simulink model "ctrl_HSMBObserver"  (R2015a)
settings: Solver=ode3  StartTime=0.0  StopTime=inf  FixedStep=0.01  RelTol=1e-3
values from neighbouring files (symbols this model uses):
  C = [C1;C2;C3;C4;C5;C6]    [initfile.m]    (also in thrustallocationQuadraticFixed.m)
  D = 3.0/100    (= 0.03)    [initfile.m]    (also in thrustallocationQuadraticFixed.m = 0.0411111111111)
  eps_c = 5    [initfile.m]
  epsilon = 0.5    [initfile.m]    (also in thrustallocationPseudo.m = u(10); thrustallocationQuadraticFixed.m = u(10))
  hd = c2d(H1,0.01,'foh')    [initfile.m]
  hd2 = c2d(H2,0.01,'zoh')    [initfile.m]
  I_s = 25000 /747225    (= 0.0334571246947)    [initfile.m]
  k_cc = 1    [initfile.m]
  K_omega = 0.3    [initfile.m]
  K_q1f = 0.0113    [initfile.m]
  K_q1r = K_q1f    (= 0.0113)    [initfile.m]
  K_q2f = 0.0117    [initfile.m]
  K_q2r = K_q2f    (= 0.0117)    [initfile.m]
  K_q3f = 0.0113    [initfile.m]
  K_q3r = K_q3f    (= 0.0113)    [initfile.m]
  K_q4f = 0.0169    [initfile.m]
  K_q4r = K_q4f    (= 0.0169)    [initfile.m]
  K_q5f = 0.0144    [initfile.m]
  K_q5r = K_q5f    (= 0.0144)    [initfile.m]
  K_q6f = 0.0168    [initfile.m]
  K_q6r = K_q6f    (= 0.0168)    [initfile.m]
  K_T1f = 0.3763    [initfile.m]
  K_T1r = K_T1f    (= 0.3763)    [initfile.m]
  K_T2f = 0.3901    [initfile.m]
  K_T2r = K_T2f    (= 0.3901)    [initfile.m]
  K_T3f = 0.3776    [initfile.m]
  K_T3r = K_T3f    (= 0.3776)    [initfile.m]
  K_T4f = 0.5641    [initfile.m]
  K_T4r = K_T4f    (= 0.5641)    [initfile.m]
  K_T5f = 0.4799    [initfile.m]
  K_T5r = K_T5f    (= 0.4799)    [initfile.m]
  K_T6f = 0.5588    [initfile.m]
  K_T6r = K_T6f    (= 0.5588)    [initfile.m]
  Kp = 3.3    [initfile.m]
  Max_Acceleration = 5    [initfile.m]
  Max_rotation = 12*sqrt(lambda)    [initfile.m]
  Max_thrust = 1.5    [initfile.m]
  Min_thrust = -0.8    [initfile.m]
  n_c = 5    [initfile.m]
  n_max = 152    [initfile.m]
  p_cc = 0.5    [initfile.m]
  pwm_thr1_backward = coeffvalues(ForceToPWM)    [initfile.m]
  pwm_thr1_forward = coeffvalues(ForceToPWM)    [initfile.m]
  pwm_thr2_backward = coeffvalues(ForceToPWM)    [initfile.m]
  pwm_thr2_forward = coeffvalues(ForceToPWM)    [initfile.m]
  pwm_thr3_backward = coeffvalues(ForceToPWM)    [initfile.m]
  pwm_thr3_forward = coeffvalues(ForceToPWM)    [initfile.m]
  pwm_thr4_backward = coeffvalues(ForceToPWM)    [initfile.m]
  pwm_thr4_forward = coeffvalues(ForceToPWM)    [initfile.m]
  pwm_thr5_backward = coeffvalues(ForceToPWM)    [initfile.m]
  pwm_thr5_forward = coeffvalues(ForceToPWM)    [initfile.m]
  pwm_thr6_backward = coeffvalues(ForceToPWM)    [initfile.m]
  pwm_thr6_forward = coeffvalues(ForceToPWM)    [initfile.m]
  Q_f0 = 0.3    [initfile.m]
  r_cc = 4    [initfile.m]
  Rho = Rho_m    (= 1000)    [initfile.m]
  ts = [-1 0]    [thrustallocationPseudo.m]    (also in thrustallocationQuadraticFixed.m)
undefined symbols (not defined in the file or in its folder): AFB, arm, Att, Control, Damping, FaultDet, Glob, Grip, IntActionType, Mass, NPO, Obs, Omg0_min, Q_max, ReferenceMdl, Sensor, Sim, SwLogic, tau, Thruster, Thruster_lock
libraries: dspmtrx3 x14, marine_gnc x11, simulink_extras x9, dspstat3 x9, simulink x9, dsparch4 x6, dspspect3 x6
(part 3 of 7)

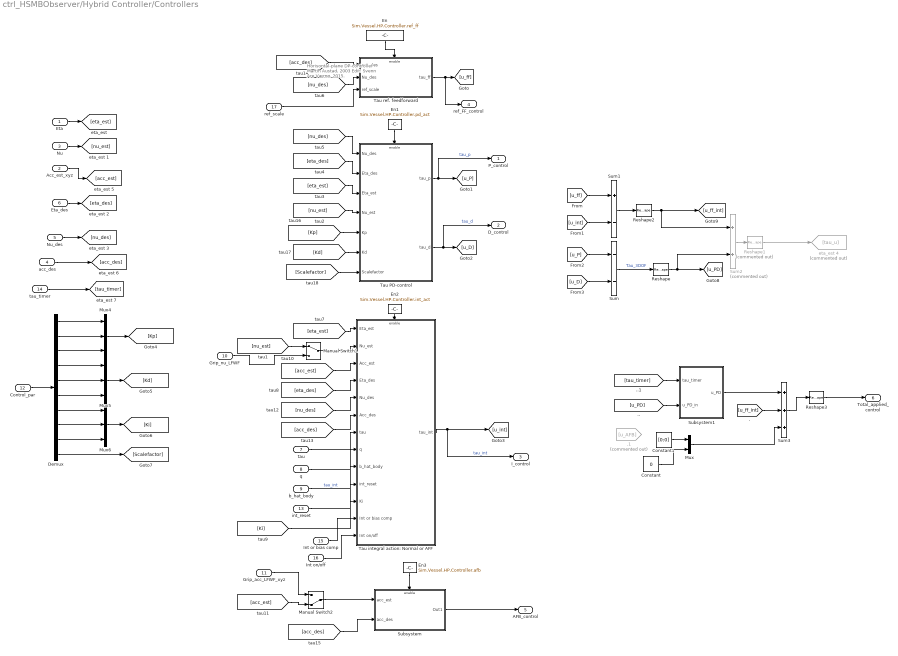
== system ctrl_HSMBObserver/Hybrid Controller/Controllers ==
  note: Horisontal-plane DP-controller
      | Martin Austad, 2003
      |
      | Edit: Svenn Are Værnø, 2015.
  Eta : Inport
  Acc_est_xyz : Inport  Port=2  PortDimensions=3
  Nu : Inport  Port=3
  acc_des : Inport  Port=4
  Nu_des : Inport  Port=5
  Eta_des : Inport  Port=6
  tau : Inport  Port=7
  q : Inport  Port=8
  b_hat_body : Inport  Port=9
  Grip_nu_LFWF : Inport  Port=10
  Grip_acc_LFWF_xyz : Inport  Port=11
  Control_par : Inport  Port=12
  int_reset : Inport  Port=13
  tau_timer : Inport  Port=14
  Int or bias comp : Inport  Port=15
  Int on/off : Inport  Port=16
  ref_scale : Inport  Port=17
  .1 : From  Commented=on  GotoTag=u_AFB
  Constant : Constant  Value=0
  Constant1 : Constant  Value=[0;0]
  Demux : Demux  Outputs=10
  En : Constant  Value=Sim.Vessel.HP.Controller.ref_ff
  En1 : Constant  Value=Sim.Vessel.HP.Controller.pd_act
  En2 : Constant  Value=Sim.Vessel.HP.Controller.int_act
  En3 : Constant  Value=Sim.Vessel.HP.Controller.afb
  Manual Switch1 : ManualSwitch
  Manual Switch2 : ManualSwitch  CurrentSetting=0
  Mux : Mux  Inputs=2
  Mux4 : Mux  Inputs=3
  Mux5 : Mux  Inputs=3
  Mux6 : Mux  Inputs=3
  Reshape : Reshape
  Reshape1 : Reshape  Commented=on
  Reshape2 : Reshape
  Reshape3 : Reshape
  Subsystem : Subsystem
  Subsystem1 : Subsystem
  Sum : Sum  Inputs=--  SaturateOnIntegerOverflow=on
  Sum1 : Sum  Inputs=+-  SaturateOnIntegerOverflow=on
  Sum2 : Sum  Commented=on  SaturateOnIntegerOverflow=on
  Sum3 : Sum  Inputs=+++  SaturateOnIntegerOverflow=on
  Tau PD-control : Subsystem
  Tau integral action: Normal or AFF : Subsystem
  Tau ref. feedforward : Subsystem
  eta_est 4 : Goto  Commented=on  GotoTag=tau_u
  P_control : Outport
  D_control : Outport  Port=2
  I_control : Outport  Port=3
  ref_FF_control : Outport  Port=4
  AFB_control : Outport  Port=5
  Total_applied_control : Outport  Port=6
  wires:
  Tau ref. feedforward/1(tau_ff) -> ref_FF_control/1, [u_ff]
  En/1 -> Tau ref. feedforward/Enable
  En2/1 -> Tau integral action: Normal or AFF/Enable
  En1/1 -> Tau PD-control/Enable
  Reshape/1 -> [u_PD], Sum2/2
  Eta/1 -> [eta_est]
  Nu/1 -> [nu_est]
  [nu_est] -> Tau PD-control/4(Nu_est)
  [eta_est] -> Tau PD-control/3(Eta_est)
  Nu_des/1 -> [nu_des]
  Eta_des/1 -> [eta_des]
  [eta_des] -> Tau PD-control/2(Eta_des)
  [nu_des] -> Tau PD-control/1(Nu_des)
  [nu_des] -> Tau ref. feedforward/2(Nu_des)
  Sum/1 -> Reshape/1  "Tau_3DOF"
  Sum2/1 -> Reshape1/1
  Reshape1/1 -> eta_est 4/1
  Reshape2/1 -> [u_ff_int], Sum2/1
  Sum1/1 -> Reshape2/1
  Tau PD-control/1(tau_p) -> P_control/1, [u_P]  "tau_p"
  Tau PD-control/2(tau_d) -> D_control/1, [u_D]  "tau_d"
  [u_ff] -> Sum1/1
  [u_int] -> Sum1/2
  [u_P] -> Sum/1
  [u_D] -> Sum/2
  Grip_nu_LFWF/1 -> Manual Switch1/2
  [nu_est] -> Manual Switch1/1
  Acc_est_xyz/1 -> [acc_est]
  En3/1 -> Subsystem/Enable
  Subsystem/1(Out1) -> AFB_control/1
  [acc_est] -> Manual Switch2/2
  Grip_acc_LFWF_xyz/1 -> Manual Switch2/1
  Manual Switch2/1 -> Subsystem/1(acc_est)
  [eta_est] -> Tau integral action: Normal or AFF/1(Eta_est)
  Manual Switch1/1 -> Tau integral action: Normal or AFF/2(Nu_est)
  [acc_est] -> Tau integral action: Normal or AFF/3(Acc_est)
  [eta_des] -> Tau integral action: Normal or AFF/4(Eta_des)
  tau/1 -> Tau integral action: Normal or AFF/7(tau)
  acc_des/1 -> [acc_des]
  Tau integral action: Normal or AFF/1(tau_int) -> I_control/1, [u_int]  "tau_int"
  [acc_des] -> Tau ref. feedforward/1(acc_des)
  [nu_des] -> Tau integral action: Normal or AFF/5(Nu_des)
  q/1 -> Tau integral action: Normal or AFF/8(q)
  b_hat_body/1 -> Tau integral action: Normal or AFF/9(b_hat_body)  "tau_int"
  [acc_des] -> Tau integral action: Normal or AFF/6(Acc_des)
  Control_par/1 -> Demux/1
  Demux/1 -> Mux4/1
  Demux/2 -> Mux4/2
  Demux/3 -> Mux4/3
  Demux/4 -> Mux5/1
  Demux/5 -> Mux5/2
  Demux/6 -> Mux5/3
  Demux/7 -> Mux6/1
  Demux/8 -> Mux6/2
  Demux/9 -> Mux6/3
  Mux4/1 -> [Kp]
  Mux5/1 -> [Kd]
  Mux6/1 -> [Ki]
  Demux/10 -> [Scalefactor]
  int_reset/1 -> Tau integral action: Normal or AFF/10(int_reset)
  [Ki] -> Tau integral action: Normal or AFF/11(Ki)
  [acc_des] -> Subsystem/2(acc_des)
  [Scalefactor] -> Tau PD-control/7(Scalefactor)
  [Kd] -> Tau PD-control/6(Kd)
  [Kp] -> Tau PD-control/5("Kp ")
  Sum3/1 -> Reshape3/1
  [u_ff_int] -> Sum3/2
  [u_PD] -> Subsystem1/2(u_PD_in)
  [tau_timer] -> Subsystem1/1(tau_timer)
  Constant/1 -> Mux/2
  Mux/1 -> Sum3/3
  Subsystem1/1(u_PD) -> Sum3/1
  Reshape3/1 -> Total_applied_control/1
  tau_timer/1 -> [tau_timer]
  Constant1/1 -> Mux/1
  Int or bias comp/1 -> Tau integral action: Normal or AFF/12(Int or bias comp)
  Int on/off/1 -> Tau integral action: Normal or AFF/13(Int on/off)
  ref_scale/1 -> Tau ref. feedforward/3(ref_scale)

== system ctrl_HSMBObserver/Hybrid Controller/Fault Detection (freeze) ==
  note: Fault detection
      | Variance testing MarReg compendium p. 153
      | SA Værnø and AH Brodtkorb fall 2015
  Eta_6DOFmeas : Inport
  Buffer : Buffer  N=FaultDet.n  V=FaultDet.ovl  ic=0.5  TreatMby1Signals=One channel
  If : If  NumInputs=2  IfExpression=u1 == u2
  If Action Subsystem : Subsystem  TreatAsAtomicUnit=on
  If Action Subsystem1 : Subsystem  TreatAsAtomicUnit=on
  Mean : dspstat3/Mean  run=off  reset_popup=None  InputProcessing=Columns as channels (frame based)  directionMode=Each column  dimension=1  treatSBRowAsCol=on  roiEnable=off  roiType=Rectangles  roiPortion=Entire ROI  roiOutput=Individual statistics for each ROI  roiFlag=off  outputDataTypeStr=Inherit: Same as accumulator  outputLastDataTypeStr=Inherit: Same as accumulator  outputMin=[]  outputMax=[]  roundingMode=Floor  overflowMode=off
  Merge : Merge
  Merge1 : Merge
  Rate Transition2 : RateTransition  Deterministic=off
  Reshape : Reshape
  Selector : Selector  InputPortWidth=6  Indices=[1]
  Unit Delay : UnitDelay  SampleTime=-1
  Zero-Order Hold3 : ZeroOrderHold  SampleTime=1/FaultDet.Fs
  fault : Outport
  pos_injection : Outport  Port=2
  wires:
  Selector/1 -> Zero-Order Hold3/1
  Eta_6DOFmeas/1 -> Selector/1
  If/1 -> If Action Subsystem/Action
  Unit Delay/1 -> If/1
  If/2 -> If Action Subsystem1/Action
  If Action Subsystem1/1(faultID) -> Merge/2
  Merge/1 -> fault/1
  If Action Subsystem/1(faultID) -> Merge/1
  Merge1/1 -> pos_injection/1
  If Action Subsystem/2(pos_inject) -> Merge1/1
  If Action Subsystem1/2(pos_inject) -> Merge1/2
  Rate Transition2/1 -> If/2, Unit Delay/1
  Buffer/1 -> Reshape/1
  Zero-Order Hold3/1 -> Buffer/1
  Reshape/1 -> Mean/1
  Mean/1 -> Rate Transition2/1

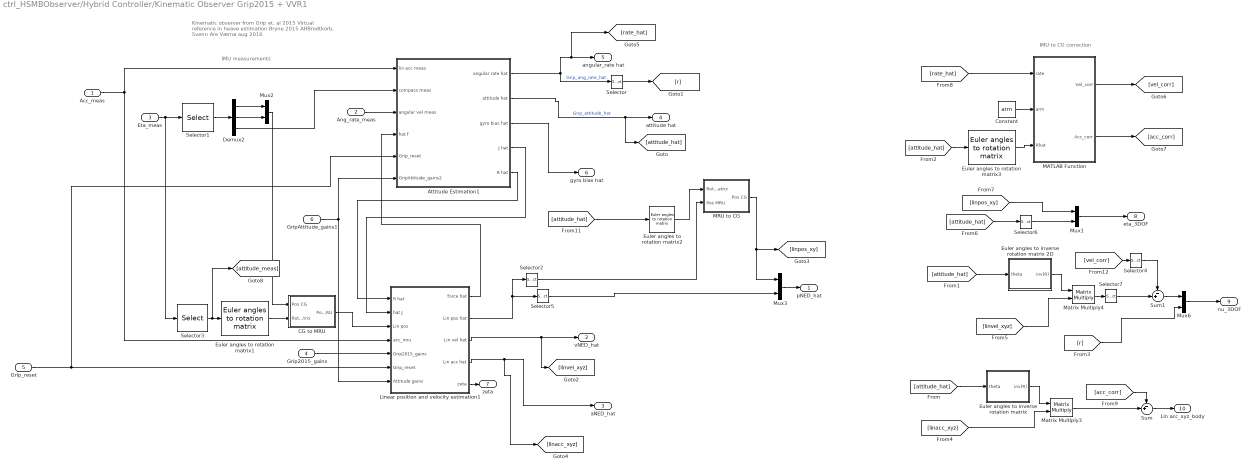
== system ctrl_HSMBObserver/Hybrid Controller/Kinematic Observer Grip2015 + VVR1 ==
  note: IMU to CG correction
  note: Kinematic observer from Grip et. al 2015
      | Virtual reference in heave estimation Bryne 2015
      | AHBrodtkorb, Svenn Are Værnø aug 2016
  note: IMU measurements
  Acc_meas : Inport
  Ang_rate_meas : Inport  Port=2
  Eta_meas : Inport  Port=3
  Grip2015_gains : Inport  Port=4
  Grip_reset : Inport  Port=5
  GripAttitude_gains1 : Inport  Port=6
  Attitude Estimation1 : Subsystem
  CG to MRU : Subsystem
  Constant : Constant  Value=arm
  Demux2 : Demux  Outputs=3
  Euler angles to inverse rotation matrix : Subsystem  AncestorBlock=|  mask(Rbn){}
      | marine_gnc/Models/ Kinematics/Euler angles to
      | inverse rotation
      | matrix
      mask help:
      | Calculate the rotation matrix from NED coordinates to Body coordinates.
      |
      | Input: Theta = [phi, theta, psi]'
      |
      | Output: inv(Rzyx) (3x3)
      mask Help:
      | Calculate the rotation matrix from NED coordinates to Body coordinates.
      | 
      | Input: Theta = [phi, theta, psi]'
      | 
      | Output: inv(Rzyx) (3x3)
  Euler angles to inverse rotation matrix 2D : Subsystem  AncestorBlock=|  mask(Rbn){}
      | marine_gnc/Models/ Kinematics/Euler angles to
      | inverse rotation
      | matrix
      mask help:
      | Calculate the rotation matrix from NED coordinates to Body coordinates.
      |
      | Input: Theta = [phi, theta, psi]'
      |
      | Output: inv(Rzyx) (3x3)
      mask Help:
      | Calculate the rotation matrix from NED coordinates to Body coordinates.
      | 
      | Input: Theta = [phi, theta, psi]'
      | 
      | Output: inv(Rzyx) (3x3)
  Euler angles to rotation matrix1 : marine_gnc/Models/ Kinematics/Euler angles to rotation matrix
  Euler angles to rotation matrix2 : marine_gnc/Models/ Kinematics/Euler angles to rotation matrix
  Euler angles to rotation matrix3 : marine_gnc/Models/ Kinematics/Euler angles to rotation matrix
  Linear position and velocity estimation1 : Subsystem
  MATLAB Function : MATLAB Function  TreatAsAtomicUnit=on
  MRU to CG : Subsystem
  Matrix Multiply3 : Product  Multiplication=Matrix(*)
  Matrix Multiply4 : Product  Multiplication=Matrix(*)
  Mux{1..3,6} (4 alike) : Mux  Inputs=2
  Selector : Selector  InputPortWidth=3  Indices=[3]
  Selector1 : Selector  InputPortWidth=6  Indices=[1 2 6]
  Selector2 : Selector  InputPortWidth=3  Indices=[1 2]
  Selector3 : Selector  InputPortWidth=6  Indices=[4 5 6]
  Selector4 : Selector  InputPortWidth=3  Indices=[1 2]
  Selector5 : Selector  InputPortWidth=3  Indices=[3]
  Selector6 : Selector  InputPortWidth=3  Indices=[3]
  Selector7 : Selector  InputPortWidth=3  Indices=[1 2]
  Sum : Sum  Inputs=-+|
  Sum1 : Sum  Inputs=-+|
  pNED_hat : Outport
  vNED_hat : Outport  Port=2
  aNED_hat : Outport  Port=3
  attitude hat : Outport  Port=4
  angular_rate hat : Outport  Port=5
  gyro bias hat : Outport  Port=6
  zeta : Outport  Port=7
  eta_3DOF : Outport  Port=8
  nu_3DOF : Outport  Port=9
  Lin acc_xyz_body : Outport  Port=10
  wires:
  Selector1/1 -> Demux2/1
  Ang_rate_meas/1 -> Attitude Estimation1/3(angular vel meas)
  Demux2/1 -> Mux2/1
  Demux2/2 -> Mux2/2
  Mux2/1 -> CG to MRU/1(Pos CG)
  Mux3/1 -> pNED_hat/1
  Linear position and velocity estimation1/4(Lin acc hat) -> [linacc_xyz], aNED_hat/1
  Linear position and velocity estimation1/3(Lin vel hat) -> [linvel_xyz], vNED_hat/1
  Linear position and velocity estimation1/2(Lin pos hat) -> Selector5/1, Selector2/1
  Selector/1 -> [r]
  Demux2/3 -> Attitude Estimation1/2(compass meas)
  MRU to CG/1(Pos CG) -> Mux3/1, [linpos_xy]
  Attitude Estimation1/2(attitude hat) -> [attitude_hat], attitude hat/1  "Grip_attitude_hat"
  Attitude Estimation1/1(angular rate hat) -> [rate_hat], angular_rate hat/1, Selector/1  "Grip_ang_rate_hat"
  Attitude Estimation1/3(gyro bias hat) -> gyro bias hat/1
  Linear position and velocity estimation1/5(zeta) -> zeta/1
  Selector5/1 -> Mux3/2
  [linacc_xyz] -> Matrix Multiply3/2
  Euler angles to inverse rotation matrix/1(inv(R)) -> Matrix Multiply3/1
  [attitude_hat] -> Euler angles to inverse rotation matrix/1(theta)
  [linvel_xyz] -> Matrix Multiply4/2
  Euler angles to inverse rotation matrix 2D/1(inv(R)) -> Matrix Multiply4/1
  [r] -> Mux6/2
  [attitude_hat] -> Euler angles to inverse rotation matrix 2D/1(theta)
  [attitude_hat] -> Selector6/1
  Selector6/1 -> Mux1/2
  [linpos_xy] -> Mux1/1
  Matrix Multiply4/1 -> Selector7/1
  Selector7/1 -> Sum1/2
  Mux6/1 -> nu_3DOF/1
  Mux1/1 -> eta_3DOF/1
  Attitude Estimation1/4(J hat) -> Linear position and velocity estimation1/2(hat J)
  Acc_meas/1 -> Attitude Estimation1/1(lin acc meas), Linear position and velocity estimation1/4(acc_imu)
  Linear position and velocity estimation1/1(force hat) -> Attitude Estimation1/4(hat f)
  Attitude Estimation1/5(R hat) -> Linear position and velocity estimation1/1(R hat)
  Grip2015_gains/1 -> Linear position and velocity estimation1/5(Grip2015_gains)
  Grip_reset/1 -> Linear position and velocity estimation1/6(Grip_reset), Attitude Estimation1/5(Grip_reset)
  Matrix Multiply3/1 -> Sum/2
  GripAttitude_gains1/1 -> Linear position and velocity estimation1/7(Attitude gains), Attitude Estimation1/6(GripAttitude_gains2)
  [attitude_hat] -> Euler angles to rotation matrix2/1
  Euler angles to rotation matrix2/1 -> MRU to CG/1(Rotation matrix)
  Selector2/1 -> MRU to CG/2(Pos MRU)
  Eta_meas/1 -> Selector3/1, Selector1/1
  Euler angles to rotation matrix1/1 -> CG to MRU/2(Rotation matrix)
  CG to MRU/1(Pos MRU) -> Linear position and velocity estimation1/3(Lin pos)
  [attitude_hat] -> Euler angles to rotation matrix3/1
  Euler angles to rotation matrix3/1 -> MATLAB Function/3(Rhat)
  Constant/1 -> MATLAB Function/2(arm)
  [rate_hat] -> MATLAB Function/1(rate)
  MATLAB Function/2(Acc_corr) -> [acc_corr]
  MATLAB Function/1(Vel_corr) -> [vel_corr]
  Sum/1 -> Lin acc_xyz_body/1
  [acc_corr] -> Sum/1
  Sum1/1 -> Mux6/1
  [vel_corr] -> Selector4/1
  Selector4/1 -> Sum1/1
  Selector3/1 -> [attitude_meas], Euler angles to rotation matrix1/1

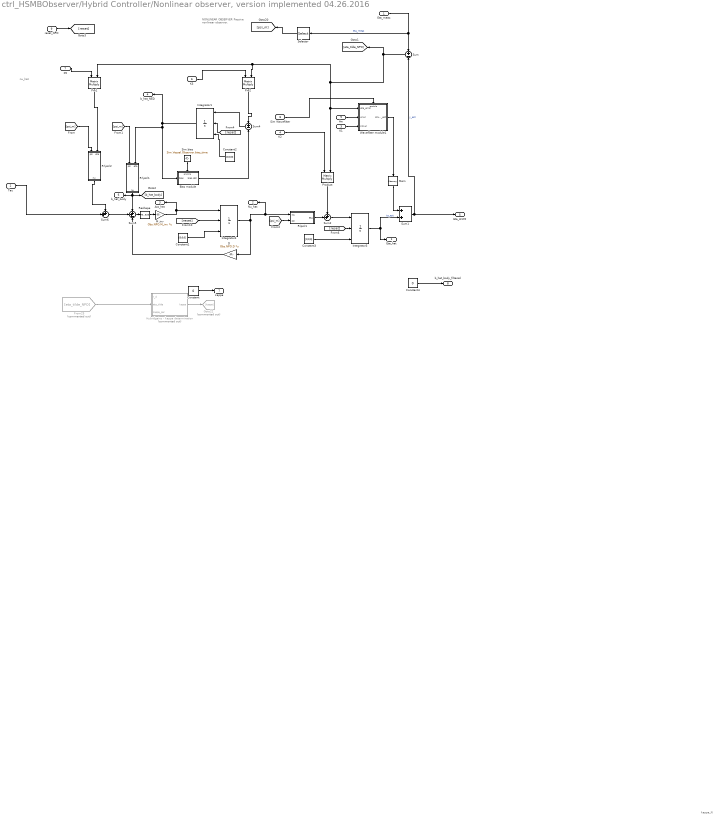
== system ctrl_HSMBObserver/Hybrid Controller/Nonlinear observer, version implemented 04.26.2016 ==
  note: NONLINEAR OBSERVER
      | Passive nonlinear observer.
  note: kappa_N
  note: nu_hat
  Eta_meas : Inport
  Tau : Inport  Port=2
  K1 : Inport  Port=3
  K2 : Inport  Port=4
  Aw : Inport  Port=5
  K3 : Inport  Port=6
  K5 : Inport  Port=7
  Sim Wavefilter : Inport  Port=8
  reset_NPO : Inport  Port=9
  Bias module : Subsystem
  Constant : Constant  Value=0
  Constant1 : Constant  Value=[0;0;0]
  Constant2 : Constant  Value=[0;0;0]
  Constant3 : Constant  Value=[0;0;0]
  Constant4 : Constant  Value=0
  D : Gain  Gain=Obs.NPO.D  Multiplication=Matrix(K*u)  SaturateOnIntegerOverflow=on  OutDataTypeStr=Inherit: Same as input  ParamDataTypeStr=Inherit: Same as input
  From25 : From  Commented=on  GotoTag=eta_tilde_NPO
  Goto22 : Goto  Commented=on  GotoTag=kappa
  Hybridgains - kappa determination : Subsystem  Commented=on
  Integrator1 : Integrator  ExternalReset=either  InitialConditionSource=external
  Integrator3 : Integrator  ExternalReset=either  InitialConditionSource=external
  Integrator4 : Integrator  ExternalReset=either  InitialConditionSource=external
  M_inv : Gain  Gain=Obs.NPO.M_inv  Multiplication=Matrix(K*u)  SaturateOnIntegerOverflow=on  OutDataTypeStr=Inherit: Same as input  ParamDataTypeStr=Inherit: Same as input
  Mem : Memory
  Pro1 : Product  Multiplication=Matrix(*)  SaturateOnIntegerOverflow=on  OutDataTypeStr=Inherit: Same as first input
  Pro2 : Product  Multiplication=Matrix(*)  SaturateOnIntegerOverflow=on  OutDataTypeStr=Inherit: Same as first input
  Product : Product  Multiplication=Matrix(*)  SaturateOnIntegerOverflow=on  OutDataTypeStr=Inherit: Same as first input
  R'(psi)1 : Subsystem
  R'(psi)2 : Subsystem
  R(psi)1 : Subsystem
  Reshape : Reshape
  Selector : Selector  InputPortWidth=3  Indices=3
  Sim.bias : Constant  Value=Sim.Vessel.Observer.bias_time
  Sum : Sum  Inputs=+-  SaturateOnIntegerOverflow=on
  Sum1 : Sum  SaturateOnIntegerOverflow=on
  Sum2 : Sum  Inputs=++|  SaturateOnIntegerOverflow=on
  Sum4 : Sum  Inputs=+-  SaturateOnIntegerOverflow=on
  Sum5 : Sum  Inputs=++-  SaturateOnIntegerOverflow=on
  Sum6 : Sum  Inputs=++|  SaturateOnIntegerOverflow=on
  Wavefilter module1 : Subsystem
  Eta_hat : Outport  InitialOutput=0
  Nu_hat : Outport  Port=2  InitialOutput=0
  Acc_hat : Outport  Port=3  InitialOutput=0
  b_hat_NED : Outport  Port=4  InitialOutput=0
  Eta_LFWF : Outport  Port=5  InitialOutput=0
  b_hat_body : Outport  Port=6  PortDimensions=3  InitialOutput=0
  kappa : Outport  Port=7  InitialOutput=0
  b_hat_body_filtered : Outport  Port=8  InitialOutput=0
  wires:
  Sim.bias/1 -> Bias module/Enable
  Bias module/1(bias.dot) -> Sum4/2
  Sim Wavefilter/1 -> Wavefilter module1/Enable
  Sum1/1 -> Sum/2, Eta_LFWF/1  "y_est"
  Mem/1 -> Sum1/1
  Selector/1 -> [psi_m]
  K1/1 -> Wavefilter module1/3(K1(w))
  Eta_meas/1 -> Selector/1, Sum/1  "eta_meas"
  M_inv/1 -> Integrator4/1, Acc_hat/1
  R'(psi)2/1(nu) -> Sum6/1
  Wavefilter module1/1(Wave_est) -> Mem/1
  Sum6/1 -> Sum5/2
  D/1 -> Sum5/3
  Integrator3/1 -> Sum1/2, Eta_hat/1  "ta_est"
  Aw/1 -> Wavefilter module1/2(A(w))
  Sum/1 -> [eta_tilde_NPO], Pro1/2, Pro2/2, Product/2, Wavefilter module1/1(eta_error)
  R'(psi)1/1(nu) -> [b_hat_body], Sum5/1, b_hat_body/1
  R(psi)1/1(Eta) -> Sum2/2
  K2/1 -> Product/1
  Tau/1 -> Sum6/2
  Pro1/1 -> R'(psi)2/2(eta)
  Pro2/1 -> Sum4/1
  Product/1 -> Sum2/1
  K5/1 -> Pro1/1
  [psi_m] -> R'(psi)2/1(psi)
  [psi_m] -> R'(psi)1/1(psi)
  [psi_m] -> R(psi)1/2(psi)
  Reshape/1 -> M_inv/1
  Sum5/1 -> Reshape/1
  From25/1 -> Hybridgains - kappa determination/2(eta_tilde)
  Hybridgains - kappa determination/1(kappa) -> Goto22/1
  reset_NPO/1 -> [reset]
  [reset] -> Integrator4/2
  Constant1/1 -> Integrator4/3
  Integrator4/1 -> Nu_hat/1, R(psi)1/1(Nu), D/1
  Sum2/1 -> Integrator3/1
  [reset] -> Integrator1/2
  Constant2/1 -> Integrator1/3
  Sum4/1 -> Integrator1/1
  Integrator1/1 -> Bias module/1(bias), R'(psi)1/2(eta), b_hat_NED/1
  [reset] -> Integrator3/2
  Constant3/1 -> Integrator3/3
  K3/1 -> Pro2/1
  Constant/1 -> kappa/1
  Constant4/1 -> b_hat_body_filtered/1

== system ctrl_HSMBObserver/Hybrid Controller/Peak Frequency FFT ==
  Eta_6DOF : Inport
  CalmWater choose PID1 : Subsystem
  Memory : Memory  X0=Control.SA.init_wp  InheritSampleTime=on
  estimate w_p : Subsystem
  hat_wp : Outport
  wires:
  Eta_6DOF/1 -> estimate w_p/1(eta_6DOF)
  Memory/1 -> hat_wp/1
  estimate w_p/1(w_p) -> CalmWater choose PID1/1(wp)
  CalmWater choose PID1/1(wp_out) -> Memory/1

== system ctrl_HSMBObserver/Hybrid Controller/Reference filter ==
  eta_d : Inport
  eta : Inport  Port=2
  PDF filter gains : Inport  Port=3
  Constant{,1..3} (4 alike) : Constant  Value=[0,0,0]
  Demux3 : Demux  Outputs=5
  Mux : Mux  Inputs=2
  Mux1 : Mux
  Scope : Scope
  Scope1 : Scope
  Subsystem : Subsystem
  Switch : Switch  Criteria=u2 > Threshold
  Switch1 : Switch  Criteria=u2 > Threshold
  Switch2 : Switch  Criteria=u2 > Threshold
  eta_c_scope1 : Scope
  eta_d1 : InportShadow
  eta_d_scpoe : Scope
  eta_f_scope : Scope
  eta_scope : Scope
  eta_tot_scop : Scope
  eta_d_f : Outport
  v_d_f : Outport  Port=2
  v_dd_f : Outport  Port=3
  wires:
  Switch/1 -> eta_tot_scop/1, eta_d_f/1
  Switch1/1 -> v_d_f/1
  Switch2/1 -> v_dd_f/1
  [enable] -> Switch/2
  [enable] -> Switch1/2
  [enable] -> Switch2/2
  eta_d/1 -> eta_d_scpoe/1, Mux/2, Switch/3
  Constant2/1 -> Switch1/3
  Constant3/1 -> Switch2/3
  eta_d1/1 -> Subsystem/1(eta_d)
  Subsystem/2(v_d_f) -> Switch1/1, Scope/1
  Subsystem/3(v_dd_f) -> Switch2/1, Scope1/1
  eta/1 -> eta_scope/1, Subsystem/2(eta1)
  Constant1/1 -> Subsystem/4(v_d)
  Constant/1 -> Subsystem/3(v_d_d)
  Mux/1 -> eta_c_scope1/1
  Subsystem/1(eta_d_f) -> Mux/1, Switch/1, eta_f_scope/1
  PDF filter gains/1 -> Demux3/1
  Demux3/1 -> Mux1/1
  Demux3/2 -> Mux1/2
  Demux3/3 -> Mux1/3
  Demux3/4 -> Mux1/4
  Mux1/1 -> [filter_gains]
  Demux3/5 -> [enable]
  [filter_gains] -> Subsystem/5(filter_gains)

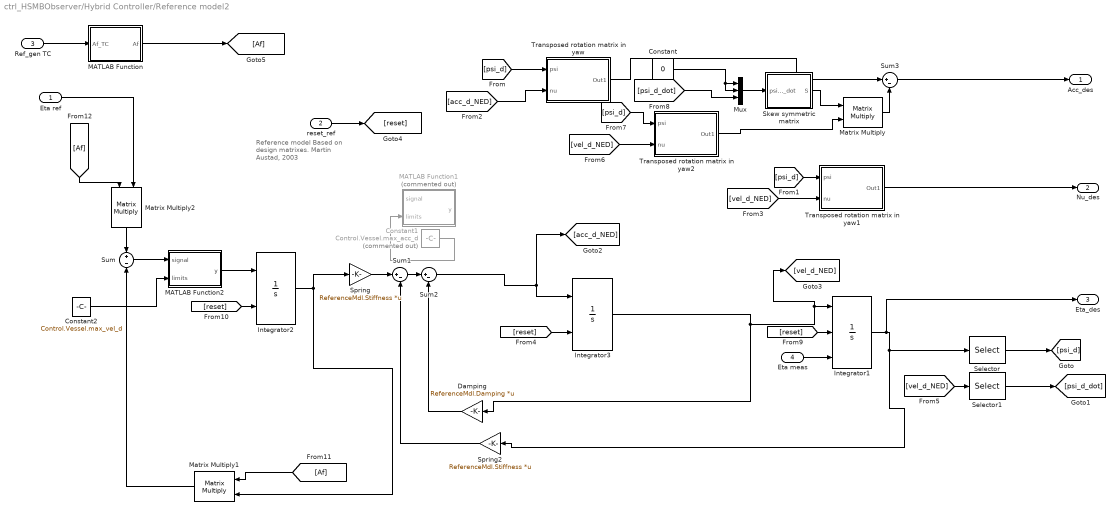
== system ctrl_HSMBObserver/Hybrid Controller/Reference model2 ==
  note: Reference model
      | Based on design matrixes.
      | Martin Austad, 2003
  Eta ref : Inport
  reset_ref : Inport  Port=2
  Ref_gen TC : Inport  Port=3
  Eta meas : Inport  Port=4
  Constant : Constant  Value=0
  Constant1 : Constant  Commented=on  Value=Control.Vessel.max_acc_d
  Constant2 : Constant  Value=Control.Vessel.max_vel_d
  Damping : Gain  Gain=ReferenceMdl.Damping  Multiplication=Matrix(K*u)  SaturateOnIntegerOverflow=on  OutDataTypeStr=Inherit: Same as input  ParamDataTypeStr=Inherit: Same as input
  Integrator1 : Integrator  ExternalReset=either  InitialConditionSource=external
  Integrator2 : Integrator  ExternalReset=either  InitialCondition=[0 0 0]
  Integrator3 : Integrator  ExternalReset=either  InitialCondition=[0 0 0]
  MATLAB Function : MATLAB Function  TreatAsAtomicUnit=on
  MATLAB Function1 : MATLAB Function  Commented=on  TreatAsAtomicUnit=on
  MATLAB Function2 : MATLAB Function  TreatAsAtomicUnit=on
  Matrix Multiply : Product  Multiplication=Matrix(*)
  Matrix Multiply1 : Product  Multiplication=Matrix(*)
  Matrix Multiply2 : Product  Multiplication=Matrix(*)
  Mux : Mux  Inputs=3
  Selector : Selector  InputPortWidth=3  Indices=[3]
  Selector1 : Selector  InputPortWidth=3  Indices=[3]
  Skew symmetric matrix : Subsystem
  Spring : Gain  Gain=ReferenceMdl.Stiffness  Multiplication=Matrix(K*u)  SaturateOnIntegerOverflow=on  OutDataTypeStr=Inherit: Same as input  ParamDataTypeStr=Inherit: Same as input
  Spring2 : Gain  Gain=ReferenceMdl.Stiffness  Multiplication=Matrix(K*u)  SaturateOnIntegerOverflow=on  OutDataTypeStr=Inherit: Same as input  ParamDataTypeStr=Inherit: Same as input
  Sum : Sum  Inputs=+|-  SaturateOnIntegerOverflow=on
  Sum1 : Sum  Inputs=|+-  SaturateOnIntegerOverflow=on
  Sum2 : Sum  Inputs=|+-  SaturateOnIntegerOverflow=on
  Sum3 : Sum  Inputs=|+-
  Transposed rotation matrix in yaw : Subsystem  AncestorBlock="marine_gnc/Models/ Kinematics/Transposed rotation  matrix in yaw"
      mask help:
      | b = R'(psi)* a
      |
      | where
      |
      | input 1:    psi
      | input 2:    a - vector dim 3
      | output 1:  b - vector dim 3
      mask Display:
      | port_label('output', 1, 'R''(psi)*v')
      | port_label('input', 1, 'psi')
      | port_label('input', 2, 'v')
  Transposed rotation matrix in yaw1 : Subsystem  AncestorBlock="marine_gnc/Models/ Kinematics/Transposed rotation  matrix in yaw"
      mask help:
      | b = R'(psi)* a
      |
      | where
      |
      | input 1:    psi
      | input 2:    a - vector dim 3
      | output 1:  b - vector dim 3
      mask Display:
      | port_label('output', 1, 'R''(psi)*v')
      | port_label('input', 1, 'psi')
      | port_label('input', 2, 'v')
  Transposed rotation matrix in yaw2 : Subsystem  AncestorBlock="marine_gnc/Models/ Kinematics/Transposed rotation  matrix in yaw"
      mask help:
      | b = R'(psi)* a
      |
      | where
      |
      | input 1:    psi
      | input 2:    a - vector dim 3
      | output 1:  b - vector dim 3
      mask Display:
      | port_label('output', 1, 'R''(psi)*v')
      | port_label('input', 1, 'psi')
      | port_label('input', 2, 'v')
  Acc_des : Outport
  Nu_des : Outport  Port=2
  Eta_des : Outport  Port=3
  wires:
  Matrix Multiply2/1 -> Sum/1
  Sum/1 -> MATLAB Function2/1(signal)
  Integrator2/1 -> Matrix Multiply1/2, Spring/1
  Matrix Multiply1/1 -> Sum/2
  Spring/1 -> Sum1/1
  Sum1/1 -> Sum2/1
  Integrator1/1 -> Spring2/1, Selector/1, Eta_des/1
  Spring2/1 -> Sum1/2
  Damping/1 -> Sum2/2
  Selector/1 -> [psi_d]
  Transposed rotation matrix in yaw/1(Out1) -> Sum3/1
  [psi_d] -> Transposed rotation matrix in yaw1/1(psi)
  [psi_d] -> Transposed rotation matrix in yaw/1(psi)
  Selector1/1 -> [psi_d_dot]
  [acc_d_NED] -> Transposed rotation matrix in yaw/2(nu)
  [vel_d_NED] -> Transposed rotation matrix in yaw1/2(nu)
  [vel_d_NED] -> Selector1/1
  [psi_d] -> Transposed rotation matrix in yaw2/1(psi)
  [vel_d_NED] -> Transposed rotation matrix in yaw2/2(nu)
  Transposed rotation matrix in yaw2/1(Out1) -> Matrix Multiply/2
  Skew symmetric matrix/1(S) -> Matrix Multiply/1
  Matrix Multiply/1 -> Sum3/2
  [psi_d_dot] -> Mux/3
  Mux/1 -> Skew symmetric matrix/1(psi_d_dot)
  Constant/1 -> Mux/1, Mux/2
  Eta ref/1 -> Matrix Multiply2/2
  reset_ref/1 -> [reset]
  [reset] -> Integrator3/2
  [reset] -> Integrator1/2
  [reset] -> Integrator2/2
  [Af] -> Matrix Multiply1/1
  Ref_gen TC/1 -> MATLAB Function/1(Af_TC)
  MATLAB Function/1(Af) -> [Af]
  Eta meas/1 -> Integrator1/3
  [Af] -> Matrix Multiply2/1
  Transposed rotation matrix in yaw1/1(Out1) -> Nu_des/1
  Sum3/1 -> Acc_des/1
  Constant1/1 -> MATLAB Function1/2(limits)
  Sum2/1 -> Integrator3/1, [acc_d_NED]
  Integrator3/1 -> [vel_d_NED], Integrator1/1, Damping/1
  Constant2/1 -> MATLAB Function2/2(limits)
  MATLAB Function2/1(y) -> Integrator2/1

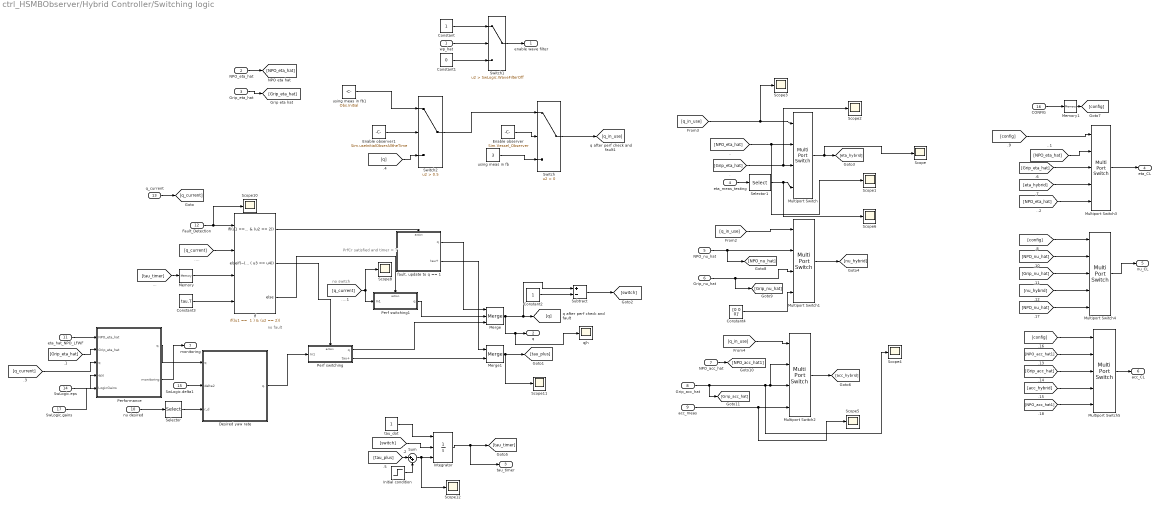
== system ctrl_HSMBObserver/Hybrid Controller/Switching logic ==
  note: PrfCr satisfied and timer = T
  note: no switch
  note: no fault
  wp_hat : Inport
  NPO_eta_hat : Inport  Port=2
  Grip_eta_hat : Inport  Port=3
  eta_meas_testing : Inport  Port=4
  NPO_nu_hat : Inport  Port=5
  Grip_nu_hat : Inport  Port=6
  NPO_acc_hat : Inport  Port=7
  Grip_acc_hat : Inport  Port=8
  acc_meas : Inport  Port=9
  nu desired : Inport  Port=10
  eta_hat_NPO_LFWF : Inport  Port=11
  Fault_Detection : Inport  Port=12
  q_current : Inport  Port=13
  SwLogic.eps : Inport  Port=14
  SwLogic.delta1 : Inport  Port=15
  CONFIG : Inport  Port=16
  SwLogic.gains : Inport  Port=17
  Constant : Constant
  Constant1 : Constant  Value=0
  Constant2 : Constant
  Constant3 : Constant  Value=tau.T
  Constant4 : Constant  Value=[0 0 0]'
  Desired yaw rate : Subsystem
  Enable observer : Constant  Value=Sim.Vessel_Observer
  Enable observer1 : Constant  Value=Sim.useInitialObserAlltheTime
  If : If  NumInputs=4  IfExpression="(u1 ==  1 ) & (u2 == 2)"  ElseIfExpressions="~(u1 ==  1) & ( u3 == u4)"
  Initial condition : Step  Before=tau.T  After=0  SampleTime=0
  Integrator : Integrator  ExternalReset=either  InitialConditionSource=external  LimitOutput=on  UpperSaturationLimit=tau.T  LowerSaturationLimit=0
  Memory : Memory
  Memory1 : Memory  X0=1
  Merge : Merge  Inputs=3
  Merge1 : Merge
  Multiport Switch : MultiPortSwitch
  Multiport Switch1 : MultiPortSwitch
  Multiport Switch2 : MultiPortSwitch
  Multiport Switch3 : MultiPortSwitch  DataPortForDefault=Additional data port  DiagnosticForDefault=None
  Multiport Switch4 : MultiPortSwitch  DataPortForDefault=Additional data port  DiagnosticForDefault=None
  Multiport Switch5 : MultiPortSwitch  DataPortForDefault=Additional data port  DiagnosticForDefault=None
  Perf switching : Subsystem  TreatAsAtomicUnit=on
  Perf switching1 : Subsystem  TreatAsAtomicUnit=on
  Performance : Subsystem
  Scope{,1..6,8,10..12} (11 alike) : Scope
      Scope settings: SaveName=ScopeData50
      Scope1 settings: SaveName=ScopeData51
      Scope10 settings: TimeRange=200  YMin=-1  YMax=1  SaveName=ScopeData153
      Scope11 settings: YMin=0  YMax=3.25e-21  SaveName=ScopeData154
      Scope12 settings: YMin=0  YMax=3.25e-21  SaveName=ScopeData163
      Scope2 settings: YMin=-0.8  YMax=0.4  SaveName=ScopeData52
      Scope3 settings: TimeRange=200  YMin=1  YMax=1  SaveName=ScopeData53
      Scope4 settings: TimeRange=1000  YMin=-0.0006  YMax=0  SaveName=ScopeData101
      Scope5 settings: YMin=-0.008  YMax=0.003  SaveName=ScopeData102
      Scope6 settings: YMin=-0.2  YMax=0  SaveName=ScopeData96
      Scope8 settings: YMin=19  YMax=21  SaveName=ScopeData151
  Selector : Selector  InputPortWidth=3  Indices=[3]
  Selector1 : Selector  InputPortWidth=6  Indices=[1 2 6]
  Subtract : Sum  Inputs=+-
  Sum : Sum  Inputs=|++
  Switch : Switch  Criteria=u2 > Threshold
  Switch1 : Switch  Criteria=u2 > Threshold  Threshold=SwLogic.WaveFilterOff  SaturateOnIntegerOverflow=on
  Switch2 : Switch  Criteria=u2 > Threshold  Threshold=0.5
  "fault, update to q == 1" : Subsystem  TreatAsAtomicUnit=on
  qjh : Scope
      settings: YMin=19  YMax=21  SaveName=ScopeData81
  tau_dot : Constant
  using meas in fb : Constant  Value=3
  using meas in fb1 : Constant  Value=Obs.Initial
  enable wave filter : Outport
  q : Outport  Port=2
  tau_timer : Outport  Port=3
  eta_CL : Outport  Port=4
  nu_CL : Outport  Port=5
  acc_CL : Outport  Port=6
  monitoring : Outport  Port=7
  wires:
  wp_hat/1 -> Switch1/2
  Constant/1 -> Switch1/1
  Constant1/1 -> Switch1/3
  Switch1/1 -> enable wave filter/1
  [NPO_eta_hat] -> Scope1/1, Multiport Switch/2
  [Grip_eta_hat] -> Scope2/1, Multiport Switch/3
  eta_meas_testing/1 -> Selector1/1
  Multiport Switch/1 -> [eta_hybrid], Scope/1
  [q_in_use] -> Multiport Switch1/1
  Multiport Switch1/1 -> [nu_hybrid]
  NPO_nu_hat/1 -> [NPO_nu_hat], Multiport Switch1/2
  Grip_nu_hat/1 -> [Grip_nu_hat], Multiport Switch1/3
  [q_in_use] -> Multiport Switch2/1
  Multiport Switch2/1 -> [acc_hybrid]
  Grip_acc_hat/1 -> [Grip_acc_hat], Scope4/1, Multiport Switch2/2, Multiport Switch2/3
  acc_meas/1 -> Multiport Switch2/4, Scope5/1
  NPO_eta_hat/1 -> [NPO_eta_hat]
  Grip_eta_hat/1 -> [Grip_eta_hat]
  eta_hat_NPO_LFWF/1 -> Performance/1(NPO_eta_hat)
  [Grip_eta_hat] -> Performance/2(Grip_eta_hat)
  Fault_Detection/1 -> Scope10/1, If/1
  If/3 -> Perf switching1/Action
  If/1 -> "fault, update to q == 1"/Action
  If/2 -> Perf switching/Action
  Enable observer/1 -> Switch/2
  using meas in fb/1 -> Switch/3
  q_current/1 -> [q_current]
  [q_current] -> If/2
  Integrator/1 -> tau_timer/1, [tau_timer]
  "fault, update to q == 1"/1(q) -> Merge/1
  Perf switching/1(q) -> Merge/3
  "fault, update to q == 1"/2(tau+) -> Merge1/1
  [tau_timer] -> Memory/1
  Constant3/1 -> If/4
  Desired yaw rate/1(q.) -> Perf switching/1(In1)
  [q_current] -> Perf switching1/1(In1), Scope8/1
  Perf switching1/1(q) -> Merge/2
  Perf switching/2(tau+) -> Merge1/2
  Merge/1 -> qjh/1, q/1, Subtract/1, [q]
  Merge1/1 -> Scope11/1, [tau_plus]
  Memory/1 -> If/3
  tau_dot/1 -> Integrator/1
  Constant2/1 -> Subtract/2
  Subtract/1 -> [switch]
  [switch] -> Integrator/2
  [tau_plus] -> Sum/1
  Initial condition/1 -> Sum/2
  Sum/1 -> Scope12/1, Integrator/3
  [q_in_use] -> Scope3/1, Multiport Switch/1
  Switch/1 -> [q_in_use]
  using meas in fb1/1 -> Switch2/1
  Enable observer1/1 -> Switch2/2
  Switch2/1 -> Switch/1
  [q] -> Switch2/3
  SwLogic.eps/1 -> Performance/4(eps)
  nu desired/1 -> Selector/1
  SwLogic.delta1/1 -> Desired yaw rate/2(delta2)
  [q_current] -> Performance/3(q)
  Performance/1(q.) -> Desired yaw rate/1(q)
  Multiport Switch3/1 -> eta_CL/1
  [NPO_eta_hat] -> Multiport Switch3/2
  [Grip_eta_hat] -> Multiport Switch3/3
  [eta_hybrid] -> Multiport Switch3/4
  Multiport Switch4/1 -> nu_CL/1
  [Grip_nu_hat] -> Multiport Switch4/3
  [NPO_nu_hat] -> Multiport Switch4/2
  [nu_hybrid] -> Multiport Switch4/4
  NPO_acc_hat/1 -> [NPO_acc_hat1]
  [Grip_acc_hat] -> Multiport Switch5/3
  [NPO_acc_hat1] -> Multiport Switch5/2
  [acc_hybrid] -> Multiport Switch5/4
  Multiport Switch5/1 -> acc_CL/1
  Selector/1 -> Desired yaw rate/3(r_d)
  [config] -> Multiport Switch3/1
  [config] -> Multiport Switch4/1
  [config] -> Multiport Switch5/1
  Memory1/1 -> [config]
  CONFIG/1 -> Memory1/1
  [NPO_eta_hat] -> Multiport Switch3/5
  [NPO_nu_hat] -> Multiport Switch4/5
  [NPO_acc_hat1] -> Multiport Switch5/5
  Constant4/1 -> Multiport Switch1/4
  Selector1/1 -> Multiport Switch/4, Scope6/1
  SwLogic.gains/1 -> Performance/5(LogicGains)
  Performance/2(monitoring) -> monitoring/1

== system ctrl_HSMBObserver/Hybrid Controller/[-inf inf] to [-pi pi] ==
  note: x
  note: r
  x [-inf inf] : Inport
  Constant : Constant  Value=2*pi
  Gain : Gain  Gain=pi  SaturateOnIntegerOverflow=on  OutDataTypeStr=Inherit: Same as input  ParamDataTypeStr=Inherit: Same as input
  Math Function : Math  Operator=rem  SaturateOnIntegerOverflow=on
  Saturation : Saturate  UpperLimit=1e10  LowerLimit=-1e10
  Sign : Signum
  Sum : Sum  Inputs=|+-  SaturateOnIntegerOverflow=on
  Sum1 : Sum  Inputs=|++  SaturateOnIntegerOverflow=on
  y [-pi pi] : Outport
  wires:
  x [-inf inf]/1 -> Saturation/1
  Sign/1 -> Gain/1
  Gain/1 -> Sum/2, Sum1/2
  Sum1/1 -> Math Function/1
  Constant/1 -> Math Function/2
  Math Function/1 -> Sum/1
  Sum/1 -> y [-pi pi]/1
  Saturation/1 -> Sum1/1, Sign/1

== system ctrl_HSMBObserver/Hybrid Controller/[-inf inf] to [-pi pi]1 ==
  note: x
  note: r
  x [-inf inf] : Inport
  Constant : Constant  Value=2*pi
  Gain : Gain  Gain=pi  SaturateOnIntegerOverflow=on  OutDataTypeStr=Inherit: Same as input  ParamDataTypeStr=Inherit: Same as input
  Math Function : Math  Operator=rem  SaturateOnIntegerOverflow=on
  Saturation : Saturate  UpperLimit=1e10  LowerLimit=-1e10
  Sign : Signum
  Sum : Sum  Inputs=|+-  SaturateOnIntegerOverflow=on
  Sum1 : Sum  Inputs=|++  SaturateOnIntegerOverflow=on
  y [-pi pi] : Outport
  wires:
  x [-inf inf]/1 -> Saturation/1
  Sign/1 -> Gain/1
  Gain/1 -> Sum/2, Sum1/2
  Sum1/1 -> Math Function/1
  Constant/1 -> Math Function/2
  Math Function/1 -> Sum/1
  Sum/1 -> y [-pi pi]/1
  Saturation/1 -> Sum1/1, Sign/1

== system ctrl_HSMBObserver/Hybrid Controller/[-inf inf] to [-pi pi]2 ==
  note: x
  note: r
  x [-inf inf] : Inport
  Constant : Constant  Value=2*pi
  Gain : Gain  Gain=pi  SaturateOnIntegerOverflow=on  OutDataTypeStr=Inherit: Same as input  ParamDataTypeStr=Inherit: Same as input
  Math Function : Math  Operator=rem  SaturateOnIntegerOverflow=on
  Saturation : Saturate  UpperLimit=1e10  LowerLimit=-1e10
  Sign : Signum
  Sum : Sum  Inputs=|+-  SaturateOnIntegerOverflow=on
  Sum1 : Sum  Inputs=|++  SaturateOnIntegerOverflow=on
  y [-pi pi] : Outport
  wires:
  x [-inf inf]/1 -> Saturation/1
  Sign/1 -> Gain/1
  Gain/1 -> Sum/2, Sum1/2
  Sum1/1 -> Math Function/1
  Constant/1 -> Math Function/2
  Math Function/1 -> Sum/1
  Sum/1 -> y [-pi pi]/1
  Saturation/1 -> Sum1/1, Sign/1

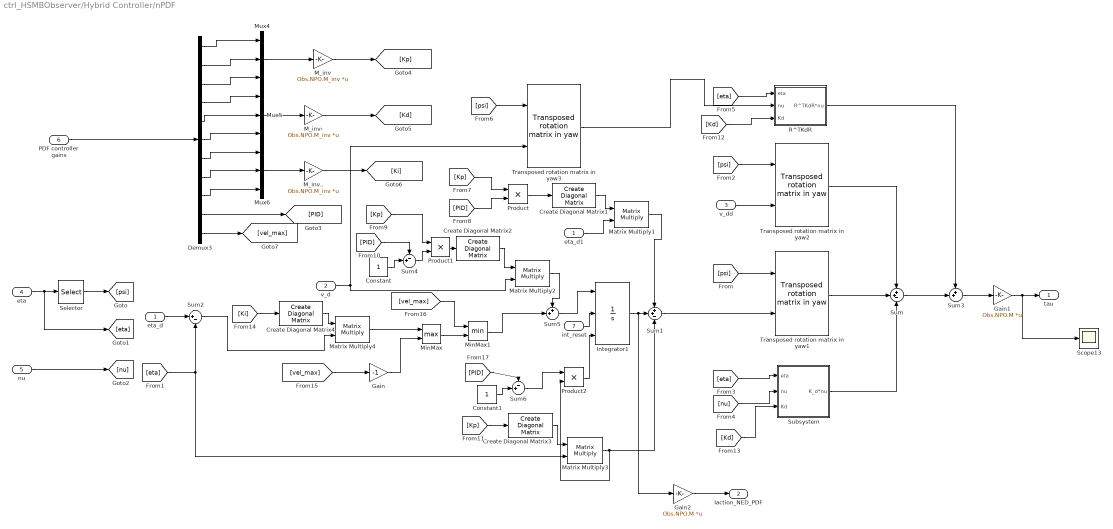
== system ctrl_HSMBObserver/Hybrid Controller/nPDF ==
  eta_d : Inport
  v_d : Inport  Port=2
  v_dd : Inport  Port=3
  eta : Inport  Port=4
  nu : Inport  Port=5
  PDF controller gains : Inport  Port=6
  int_reset : Inport  Port=7
  Constant : Constant
  Constant1 : Constant
  Create Diagonal Matrix{1..4} (4 alike) : dspmtrx3/Create Diagonal Matrix
  Demux3 : Demux  Outputs=11
  Gain : Gain  Gain=-1
  Gain1 : Gain  Gain=Obs.NPO.M  Multiplication=Matrix(K*u)
  Gain2 : Gain  Gain=Obs.NPO.M  Multiplication=Matrix(K*u)
  Integrator1 : Integrator  ExternalReset=either  InitialConditionSource=external
  M_inv : Gain  Gain=Obs.NPO.M_inv  Multiplication=Matrix(K*u)
  M_inv- : Gain  Gain=Obs.NPO.M_inv  Multiplication=Matrix(K*u)
  M_inv.. : Gain  Gain=Obs.NPO.M_inv  Multiplication=Matrix(K*u)
  Matrix Multiply{1..4} (4 alike) : Product  Multiplication=Matrix(*)
  MinMax : MinMax  Function=max  Inputs=2
  MinMax1 : MinMax  Inputs=2
  Mux4 : Mux  Inputs=3
  Mux5 : Mux  Inputs=3
  Mux6 : Mux  Inputs=3
  Product : Product
  Product1 : Product
  Product2 : Product
  R^TKdR : Subsystem
  Scope13 : Scope
  Selector : Selector  InputPortWidth=3  Indices=3
  Subsystem : Subsystem
  Sum : Sum  Inputs=++-
  Sum1 : Sum  Inputs=++-
  Sum2 : Sum  Inputs=|+-
  Sum3 : Sum  Inputs=++|
  Sum4 : Sum  Inputs=-+|
  Sum5 : Sum  Inputs=++|
  Sum6 : Sum  Inputs=-+|
  Transposed rotation matrix in yaw1 : marine_gnc/Models/ Kinematics/Transposed rotation  matrix in yaw
  Transposed rotation matrix in yaw2 : marine_gnc/Models/ Kinematics/Transposed rotation  matrix in yaw
  Transposed rotation matrix in yaw3 : marine_gnc/Models/ Kinematics/Transposed rotation  matrix in yaw
  eta_d1 : InportShadow
  tau : Outport
  Iaction_NED_PDF : Outport  Port=2
  wires:
  Sum2/1 -> Matrix Multiply4/2
  eta_d/1 -> Sum2/1
  Sum3/1 -> Gain1/1
  Sum1/1 -> Transposed rotation matrix in yaw1/2
  eta/1 -> [eta], Selector/1
  Selector/1 -> [psi]
  v_d/1 -> Matrix Multiply2/2, Transposed rotation matrix in yaw3/2
  [psi] -> Transposed rotation matrix in yaw1/1
  Transposed rotation matrix in yaw1/1 -> Sum/2
  v_dd/1 -> Transposed rotation matrix in yaw2/2
  Transposed rotation matrix in yaw2/1 -> Sum/1
  [psi] -> Transposed rotation matrix in yaw2/1
  [eta] -> Subsystem/1(eta)
  [nu] -> Subsystem/2(nu)
  [eta] -> R^TKdR/1(eta)
  [psi] -> Transposed rotation matrix in yaw3/1
  Transposed rotation matrix in yaw3/1 -> R^TKdR/2(nu)
  R^TKdR/1(R^TKdR*nu) -> Sum3/1
  Sum/1 -> Sum3/2
  Gain1/1 -> Scope13/1, tau/1
  Sum5/1 -> Integrator1/1
  MinMax1/1 -> Sum5/2
  eta_d1/1 -> Matrix Multiply1/2
  Matrix Multiply1/1 -> Sum1/1
  Matrix Multiply3/1 -> Product2/2, Sum1/3
  Matrix Multiply2/1 -> Sum5/1
  [eta] -> Matrix Multiply3/2, Sum2/2
  Integrator1/1 -> Gain2/1, Sum1/2
  Subsystem/1(K_d*nu) -> Sum/3
  nu/1 -> [nu]
  Demux3/1 -> Mux4/1
  Demux3/2 -> Mux4/2
  Demux3/3 -> Mux4/3
  Demux3/4 -> Mux5/1
  Demux3/5 -> Mux5/2
  Demux3/6 -> Mux5/3
  Demux3/7 -> Mux6/1
  Demux3/8 -> Mux6/2
  Demux3/9 -> Mux6/3
  Mux4/1 -> M_inv/1
  Mux5/1 -> M_inv-/1
  Mux6/1 -> M_inv../1
  PDF controller gains/1 -> Demux3/1
  Create Diagonal Matrix1/1 -> Matrix Multiply1/1
  Product/1 -> Create Diagonal Matrix1/1
  [Kp] -> Product/1
  [PID] -> Product/2
  Demux3/10 -> [PID]
  [Kp] -> Product1/1
  Constant/1 -> Sum4/2
  [PID] -> Sum4/1
  Sum4/1 -> Product1/2
  Product1/1 -> Create Diagonal Matrix2/1
  Create Diagonal Matrix2/1 -> Matrix Multiply2/1
  Create Diagonal Matrix3/1 -> Matrix Multiply3/1
  [Kp] -> Create Diagonal Matrix3/1
  int_reset/1 -> Integrator1/2
  Product2/1 -> Integrator1/3
  [Kd] -> R^TKdR/3(Kd)
  [Kd] -> Subsystem/3(Kd)
  Create Diagonal Matrix4/1 -> Matrix Multiply4/1
  [Ki] -> Create Diagonal Matrix4/1
  MinMax/1 -> MinMax1/2
  Matrix Multiply4/1 -> MinMax/1
  Demux3/11 -> [vel_max]
  [vel_max] -> Gain/1
  Gain/1 -> MinMax/2
  [vel_max] -> MinMax1/1
  M_inv/1 -> [Kp]
  M_inv-/1 -> [Kd]
  M_inv../1 -> [Ki]
  Gain2/1 -> Iaction_NED_PDF/1
  Constant1/1 -> Sum6/2
  [PID] -> Sum6/1
  Sum6/1 -> Product2/1

== system ctrl_HSMBObserver/Thrust allocation1/Optimal angle path and constraints on rotation speed ==
  Desired Angle : Inport  Partition=on  PartitionDimension=1  PartitionWidth=1
  "initial angle " : Inport  Port=2  Partition=on  PartitionDimension=1  PartitionWidth=1
  reset : Inport  Port=3  Partition=on  PartitionDimension=1  PartitionWidth=1
  Degrees to Radians : simulink_extras/Transformations/Degrees to Radians
  Delay : Delay  DelayLength=1  InitialCondition=0
  Discrete-Time Integrator : DiscreteIntegrator  ExternalReset=either  InitialConditionSource=external  InitialConditionSetting=State (most efficient)  SampleTime=0.01
  Ensuring angle is [-pi pi] : MATLAB Function  TreatAsAtomicUnit=on
  For Each : ForEach  DisableCoverage=on  IndexMode=One-based
  MATLAB Function1 : MATLAB Function  TreatAsAtomicUnit=on
  Max Rotation Rate : Saturate  UpperLimit=Max_rotation  LowerLimit=-Max_rotation
  commanded Angle : Outport  ConcatenationDimension=1
  wires:
  Degrees to Radians/1 -> Ensuring angle is [-pi pi]/1(angle)
  Ensuring angle is [-pi pi]/1(y) -> commanded Angle/1
  Discrete-Time Integrator/1 -> Degrees to Radians/1, Delay/1  "angle"
  "initial angle "/1 -> Discrete-Time Integrator/3
  Max Rotation Rate/1 -> Discrete-Time Integrator/1
  MATLAB Function1/1(psi_D) -> Max Rotation Rate/1
  Desired Angle/1 -> MATLAB Function1/1(desired)
  reset/1 -> Discrete-Time Integrator/2
  Delay/1 -> MATLAB Function1/2(actual)

== system ctrl_HSMBObserver/Thruster control /Subsystem1 ==
  Calculated angles : Inport
  Demux : Demux  Outputs=6
  Mux : Mux  Inputs=6
  Saturation {1..6} (6 alike) : Saturate  UpperLimit=pi  LowerLimit=-pi
  Commanded angles : Outport
  wires:
  Calculated angles/1 -> Demux/1
  Demux/1 -> Saturation 1/1
  Demux/2 -> Saturation 2/1
  Demux/3 -> Saturation 3/1
  Demux/4 -> Saturation 4/1
  Demux/5 -> Saturation 5/1
  Demux/6 -> Saturation 6/1
  Mux/1 -> Commanded angles/1
  Saturation 1/1 -> Mux/1
  Saturation 6/1 -> Mux/6
  Saturation 5/1 -> Mux/5
  Saturation 2/1 -> Mux/2
  Saturation 3/1 -> Mux/3
  Saturation 4/1 -> Mux/4
